simulink model "AtomicVsNonAtomicSubsys"  (R2020a)
settings: Solver=FixedStepDiscrete  StartTime=0.0  StopTime=10.0  FixedStep=1  RelTol=1e-3
settings Model: OrderedModelArguments=off  Creator=ashok  LastModifiedBy=ashok
settings OptimizationCC: DefaultParameterBehavior=Inlined  EnhancedBackFolding=on  PassReuseOutputArgsAs=Individual arguments  ZeroExternalMemoryAtStartup=off  ZeroInternalMemoryAtStartup=off  OptimizeBlockOrder=speed  DifferentSizesBufferReuse=on  OptimizationCustomize=off  EfficientTunableParamExpr=on
settings DebuggingCC: ParameterTunabilityLossMsg=error
settings SFSimCC: MATLABDynamicMemAlloc=off
settings RTWCC: SystemTargetFile=ert.tlc  GenCodeOnly=on  TemplateMakefile=ert_default_tmf
settings CodeAppCC: ForceParamTrailComments=on  IgnoreCustomStorageClasses=off  OperatorAnnotations=on  SimulinkDataObjDesc=on  SFDataObjDesc=on  InsertBlockDesc=on
settings ERTTargetCC: TargetLangStandard=C99 (ISO)  GenerateSampleERTMain=on  InlinedParameterPlacement=NonHierarchical  ERTCustomFileTemplate=example_file_process.tlc
settings ConfigComp: PSAutoStubLUT=on

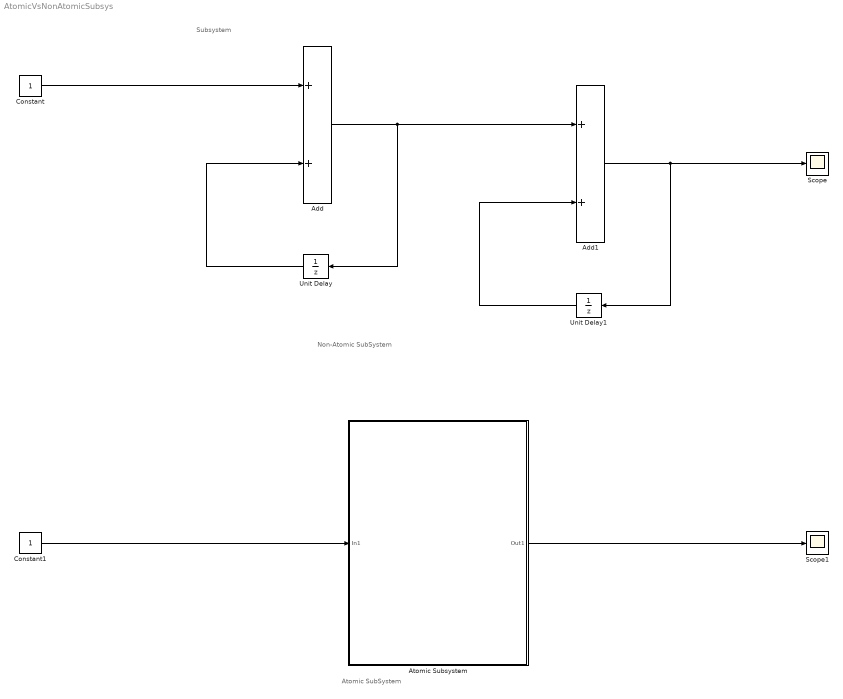
== system AtomicVsNonAtomicSubsys ==
  note: Non-Atomic SubSystem
  note: Subsystem
  note: Atomic SubSystem
  Add : Sum
  Add1 : Sum
  Atomic Subsystem : Subsystem  TreatAsAtomicUnit=on
  Constant : Constant
  Constant1 : Constant
  Scope : Scope
  Scope1 : Scope
  Unit Delay : UnitDelay  SampleTime=-1  HasFrameUpgradeWarning=on
  Unit Delay1 : UnitDelay  SampleTime=-1  HasFrameUpgradeWarning=on
  wires:
  Add1/1 -> Scope/1, Unit Delay1/1
  Constant/1 -> Add/1
  Unit Delay1/1 -> Add1/2
  Add/1 -> Add1/1, Unit Delay/1
  Unit Delay/1 -> Add/2
  Constant1/1 -> Atomic Subsystem/1(In1)
  Atomic Subsystem/1(Out1) -> Scope1/1

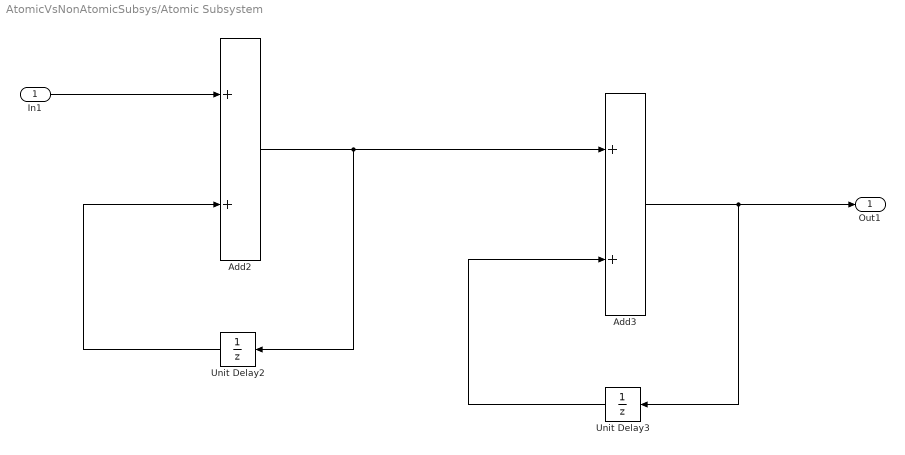
== system AtomicVsNonAtomicSubsys/Atomic Subsystem ==
  In1 : Inport
  Add2 : Sum
  Add3 : Sum
  Unit Delay2 : UnitDelay  SampleTime=-1  HasFrameUpgradeWarning=on
  Unit Delay3 : UnitDelay  SampleTime=-1  HasFrameUpgradeWarning=on
  Out1 : Outport
  wires:
  Add2/1 -> Add3/1, Unit Delay2/1
  Unit Delay2/1 -> Add2/2
  Add3/1 -> Out1/1, Unit Delay3/1
  Unit Delay3/1 -> Add3/2
  In1/1 -> Add2/1
